simulink model "HighpassFilterModel"  (R2019b)
settings: Solver=VariableStepAuto  StartTime=0.0  StopTime=10.0  RelTol=1e-3
settings Model: Creator=ip  LastModifiedBy=ip

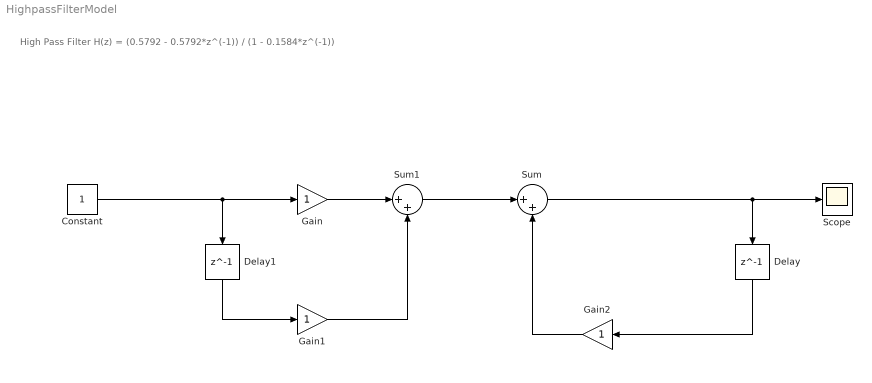
== system HighpassFilterModel ==
  note: High Pass Filter
      |
      | H(z) = (0.5792 - 0.5792*z^(-1)) / (1 - 0.1584*z^(-1))
  Constant : Constant
  Delay : Delay  DelayLength=1
  Delay1 : Delay  DelayLength=1
  Gain : Gain
  Gain1 : Gain
  Gain2 : Gain
  Scope : Scope
  Sum : Sum  Inputs=|++
  Sum1 : Sum  Inputs=|++
  wires:
  Constant/1 -> Gain/1, Delay1/1
  Gain/1 -> Sum1/1
  Sum1/1 -> Sum/1
  Sum/1 -> Delay/1, Scope/1
  Delay/1 -> Gain2/1
  Gain2/1 -> Sum/2
  Delay1/1 -> Gain1/1
  Gain1/1 -> Sum1/2
